simulink model "MCity_cs"  (Simulink 8.9)
settings: Solver=ode5  StartTime=0.0  StopTime=2.95  FixedStep=1/200  RelTol=1e-3
PreLoadFcn:
  | check_NUTS_defined;
  | 
  | assignin('base',['model_closed_' bdroot],false);
InitFcn:
  | PreScanExperimentInitFcn(bdroot)
StopFcn:
  | PreScanExperimentStopFcn(bdroot)
values from neighbouring files (symbols this model uses):
  d_offset = -18.15    [monocityTestLeftTurn.mat]    (also in simulation_leftTurn_PreScan.m = dl/vl*vh - 43 + R)
  vh = vhN(i)    [evaluation_leftTurn_Simulink.m]    (also in generate_leftTurn_accelerated.m = ones(N,1); generate_leftTurn_naturalistic.m = ones(N,1); monocityTestLeftTurn.mat = 30; monotonicityTest.m = i)
  vl = vlN(i)    [evaluation_leftTurn_Simulink.m]    (also in generate_leftTurn_accelerated.m = ones(N,1); generate_leftTurn_naturalistic.m = ones(N,1); monocityTestLeftTurn.mat = 60; monotonicityTest.m = j)
undefined symbols (not defined in the file or in its folder): DiscIntNeverNeededParam, warningInitialVelocity, x0
libraries: simulink x73, PreScanSimulinkLibrary x14, simulink_extras x10, PreScanUsefulBlocks x4
(part 11 of 11)

== matlab function BMW_Z3_1/MATLAB Function ==
  data: x_av input double; range output double; y_av input double; h_av_in input double; x_t input double; y_t input double; theta_worldCoordinates output double; h_av output double; theta_sensorCoordinates output double
function [range,theta_worldCoordinates,h_av,theta_sensorCoordinates] = fcn(x_av,y_av,h_av_in,x_t,y_t)
    
    range = norm([x_av-x_t,y_av-y_t]);
    theta_worldCoordinates = atan2(x_t-x_av,y_t-y_av)*180/pi;
    h_av = h_av_in;
    theta_sensorCoordinates = ((theta_worldCoordinates-h_av)*pi/180);
    theta_sensorCoordinates = mod(theta_sensorCoordinates + pi,2*pi) - pi;
    theta_sensorCoordinates = theta_sensorCoordinates/pi*180;
end

== matlab function BMW_Z3_1/Subsystem/PreBraking Model/Straight road segment/Relative velocity1/Translation ==
  data: v input double; xpd input double; xp_dot output double; TISdet parameter double
function xp_dot = trans(v, xpd, TISdet)
%#codegen
%Translation of the value

xp_dot = xpd;
for i = 1 : TISdet(1)
    if xpd(i) == v
        xp_dot(i) = 0;
    end
end
end

== matlab function BMW_Z3_1/Subsystem/PreBraking Model/Straight road segment/Relative velocity1/Embedded MATLAB Function1 ==
  settings: updateMethod=DISCRETE
  data: r input double; yp2 output double; yp1 input double; K1 input double; K2 output double; TISdet parameter double; TISMaxRange parameter double
function [yp2, K2] = modif(r, yp1, K1, TISdet, TISMaxRange)
%#codegen
% Interpolating yp value.

K2 = K1;
yp2 = yp1;

d = 50;

% Adding point
for i = 1 : TISdet(1)
   if r(i) ~= TISMaxRange(1)
      K2(i,1:d-1) = K2(i,2:d);
      K2(i,d) = yp1(i);
   end
end

% Choosing what to take
for i = 1 : TISdet(1)
    s = 0;
    suma = 0;
    for j = 1 : 50
        if K2(i,j) ~= 0
            suma = suma + K2(i,j);
            s = s + 1;
        end
    end
    yp2(i) = suma/s;
end

% Returning, if object is not detected
for i = 1: TISdet(1)
    if r(i) == TISMaxRange(1) && yp1(i) == 0
        K2(i,:,:) = zeros(d,1);
        yp2(i) = 0;
    end    
end

== matlab function Audi_A8_1/PathFollower_Preview_1/LateralController/Calculate delta steering error/eml_delta_steering_error ==
  data: v_x_vehicle input double; v_x_vehicle_Min input double; t_Preview_LatCtrl input double; delta_steeringwheeltotal output double; v_y_vehicle input double; yawrate_vehicle input double; CorneringStiffness_Tyres_Front input double; CorneringStiffness_Tyres_Rear input double; m_vehicle_total input double; inertia_z_vehicle_total input double; e_Lat input double size=10; Pos_x_CoG_Vehicle input double; wheelbase input double; RefreshCounter parameter double
function delta_steeringwheeltotal = eml_delta_steering_error(v_x_vehicle,v_x_vehicle_Min,t_Preview_LatCtrl,v_y_vehicle,yawrate_vehicle,CorneringStiffness_Tyres_Front,CorneringStiffness_Tyres_Rear,m_vehicle_total,inertia_z_vehicle_total,e_Lat,Pos_x_CoG_Vehicle,wheelbase,RefreshCounter)

delta_steeringwheeltotal = emlfcn_delta_steering_error(v_x_vehicle,v_x_vehicle_Min,t_Preview_LatCtrl,v_y_vehicle,yawrate_vehicle,CorneringStiffness_Tyres_Front,CorneringStiffness_Tyres_Rear,m_vehicle_total,inertia_z_vehicle_total,e_Lat,Pos_x_CoG_Vehicle,wheelbase,RefreshCounter);

% end function

== matlab function BMW_Z3_1/Subsystem/PreBraking Model/Straight road segment/Relative velocity2/Embedded MATLAB Function1 ==
  data: r input double; yp2 output double; yp1 input double; K1 input double; K2 output double; TISdet parameter double; TISMaxRange parameter double
function [yp2, K2] = modif(r, yp1, K1, TISdet, TISMaxRange)
%#codegen
% Interpolating yp value.

K2 = K1;
yp2 = yp1;

d = 50;

% Adding point
for i = 1 : TISdet(2)
   if r(i) ~= 5*TISMaxRange(2) 
      K2(i,1:d-1) = K2(i,2:d);
      K2(i,d) = yp1(i);
   end
end

% Choosing what to take
for i = 1 : TISdet(2)
    s = 0;
    suma = 0;
    for j = 1 : 50
        if K2(i,j) ~= 0
            suma = suma + K2(i,j);
            s = s + 1;
        end
    end
    yp2(i) = suma/s;
end

% Returning, if object is not detected
for i = 1: TISdet(2)
    if r(i) == 30 && yp1(i) == 0
        K2(i,:,:) = zeros(d,1);
        yp2(i) = 0;
    end    
end

== matlab function BMW_Z3_1/Subsystem/PreBraking Model/Straight road segment/Relative velocity2/Translation ==
  data: v input double; xpd input double; xp_dot output double; TISdet parameter double
function xp_dot = trans(v, xpd, TISdet)
%#codegen
%Translation of the value

xp_dot = xpd;
for i = 1 : TISdet(2)
    if xpd(i) == v
        xp_dot(i) =0;
    end
end
end

== matlab function BMW_Z3_1/Subsystem/PreBraking Model/TIS1sorting_fun/Embedded MATLAB Function ==
  data: range input double; indx input double; RANGE output double; TISdet parameter double
function RANGE = dis(range, indx, TISdet)
%#codegen

RANGE = zeros(TISdet(1),1);
for i = 1 : length(indx)
    if indx(i) ~= 0
        RANGE(i) = range(indx(i));
    else
        RANGE(i) = 0;
    end
end

== matlab function BMW_Z3_1/Subsystem/PreBraking Model/Straight road segment/THETA Derivative1/Deriv correction ==
  data: th input double; thp input double; thd input double; th_dot output double; TISdet parameter double
function th_dot = stopping(th, thp, thd, TISdet)
%#codegen
% Stopping if nothing is detected.

th_dot = thd;
for i = 1 : TISdet(2)
    if (th(i)==0 && thp(i)~=0) || (th(i)~=0 && thp(i)==0)
        th_dot(i) = 0;
    end
end
end

== matlab function BMW_Z3_1/Subsystem/PreBraking Model/Straight road segment/THETA Derivative2/Deriv correction ==
  data: th input double; thp input double; thd input double; th_dot output double; TISdet parameter double
function th_dot = stopping(th, thp, thd, TISdet)
%#codegen
% Stopping if nothing is detected.

th_dot = thd;
for i = 1 : TISdet(1)
    if (th(i)==0 && thp(i)~=0) || (th(i)~=0 && thp(i)==0)
        th_dot(i) = 0;
    end
end
end

== matlab function BMW_Z3_1/Subsystem/PreBraking Model/Straight road segment/THETA Derivative2/Theta extrapolation ==
  data: r input double; th1 input double; th2 output double; thd input double; time input double; K1 input double; K2 output double; TISdet parameter double; TISMaxRange parameter double
function [th2, K2] = modif(r, th1, thd, time, K1, TISdet, TISMaxRange)
%#codegen
% Interpolating theta value.

K2 = K1;
th2 = th1;

d = 10;

% Finding points used in interpolation/extrapolation.
for i = 1 : TISdet(1)
    if thd(i) ~= 0
        K2(i,1:d-1,:) = K2(i,2:d,:);
        K2(i,  d,1) = time;
        K2(i,  d,2) = th1(i);
    end
end

% Extrapolation
for i = 1 : TISdet(1)
    j = 1;
    while j < d+1 && K2(i,j,1) == 0
        j = j + 1;
    end
    
    if j > d-2
        th2(i) = th1(i);
    else
        th2(i) = interp1(K2(i,d-2:d,1),K2(i,d-2:d,2),time,'linear','extrap');
    end
end

% Returning, if object is not detected
for i = 1: TISdet(1)
    if r(i) == TISMaxRange(1) && th1(i) == 0
        K2(i,:,:) = zeros(d,2);
        th2(i) = 0;
    end    
end

end

== matlab function BMW_Z3_1/Subsystem/PreBraking Model/Straight road segment/THETA Derivative1/Theta extrapolation ==
  data: r input double; th1 input double; th2 output double; thd input double; time input double; K1 input double; K2 output double; TISdet parameter double; TISMaxRange parameter double
function [th2, K2] = modif(r, th1, thd, time, K1, TISdet, TISMaxRange)
%#codegen
% Interpolating theta value.

K2 = K1;
th2 = th1;

d = 10;

% Finding points used in interpolation/extrapolation.
for i = 1 : TISdet(2)
    if thd(i) ~= 0
        K2(i,1:d-1,:) = K2(i,2:d,:);
        K2(i,  d,1) = time;
        K2(i,  d,2) = th1(i);
    end
end

% Extrapolation
for i = 1 : TISdet(2)
    j = 1;
    while j < d+1 && K2(i,j,1) == 0
        j = j + 1;
    end
    
    if j > d-2
        th2(i) = th1(i);
    else
        th2(i) = interp1(K2(i,d-2:d,1),K2(i,d-2:d,2),time,'linear','extrap');
    end
end

% Returning, if object is not detected
for i = 1: TISdet(2)
    if r(i) == 5*TISMaxRange(2) && th1(i) == 0
        K2(i,:,:) = zeros(d,2);
        th2(i) = 0;
    end    
end

end

== matlab function BMW_Z3_1/Subsystem/PreBraking Model/Bend road segment/T2.6/median filter/median function ==
  data: u input double; y output double; TISdet parameter double
function y = fcn(u, TISdet)
%#codegen


nr = 1;
y = zeros(TISdet(nr),1,'int16');

for kk = 1 : TISdet(nr)
    z = 0;
    w = 0;
    for ii = 0 : 2
        if u(TISdet(nr)*ii+kk) == true
            w = w + 1;
        else
            z = z + 1;
        end
    end
    
    if w > z
        y(kk) = int16(1);
    end
end

end

== matlab function BMW_Z3_1/Subsystem/PreBraking Model/Bend road segment/T1.6/median filter/median function ==
  data: u input double; y output double; TISdet parameter double
function y = fcn(u, TISdet)
%#codegen


nr = 1;
y = zeros(TISdet(nr),1,'int16');

for kk = 1 : TISdet(nr)
    z = 0;
    w = 0;
    for ii = 0 : 2
        if u(TISdet(nr)*ii+kk) == true
            w = w + 1;
        else
            z = z + 1;
        end
    end
    
    if w > z
        y(kk) = int16(1);
    end
end

end

== matlab function BMW_Z3_1/Subsystem/PreBraking Model/Straight road segment/T1.6/median filter/median function ==
  data: u input double; y output double; TISdet parameter double
function y = fcn(u, TISdet)
%#codegen


nr = 1;
y = zeros(TISdet(nr),1,'int16');

for kk = 1 : TISdet(nr)
    z = 0;
    w = 0;
    for ii = 0 : 2
        if u(TISdet(nr)*ii+kk) == true
            w = w + 1;
        else
            z = z + 1;
        end
    end
    
    if w > z
        y(kk) = int16(1);
    end
end

end

== matlab function BMW_Z3_1/Subsystem/PreBraking Model/Straight road segment/T2.6/median filter/median function ==
  data: u input double; y output double; TISdet parameter double
function y = fcn(u, TISdet)
%#codegen


nr = 1;
y = zeros(TISdet(nr),1,'int16');

for kk = 1 : TISdet(nr)
    z = 0;
    w = 0;
    for ii = 0 : 2
        if u(TISdet(nr)*ii+kk) == true
            w = w + 1;
        else
            z = z + 1;
        end
    end
    
    if w > z
        y(kk) = int16(1);
    end
end

end

== matlab function BMW_Z3_1/Subsystem/PreBraking Model/TIS1sorting_fun/Embedded MATLAB Function1 ==
  data: indx input double; THETA output double; theta input double; TISdet parameter double
function THETA = ang(indx, theta, TISdet)
%#codegen

THETA = zeros(TISdet(1),1);
for i = 1 : length(indx)
    if indx(i) ~= 0
        THETA(i) = theta(indx(i));
    else
        THETA(i) = 0;
    end
end

== matlab function BMW_Z3_1/Subsystem/PreBraking Model/TIS1sorting_fun/Embedded MATLAB Function2 ==
  data: indx input double; RANGEDOT output double; rangedot input double; TISdet parameter double
function RANGEDOT = vel(indx, rangedot, TISdet)
%#codegen

RANGEDOT = zeros(TISdet(1),1);
for i = 1 : length(indx)
    if indx(i) ~= 0
        RANGEDOT(i) = rangedot(indx(i));
    else
        RANGEDOT(i) = 0;
    end
end

== matlab function BMW_Z3_1/Subsystem/PreBraking Model/TIS1sorting_fun/MATLAB Function ==
  data: indxp input double; indx output double; range input double; TISdet parameter double
function indx = sorts(indxp, range, TISdet)
%#codegen

size = TISdet(1);

indx = indxp;

for i = 1 : size
    if ( indx(i) ~= 0 ) && ( range(i) == 0)
        indx(i) = 0;
    end
end

for i = 1 : size
    if indx(i) ~= 0
        range(i) = 0;
    end
end

for i = 1 : size
    if range(i) ~= 0
       j = 1;
       while( indx(j) )
           j = j + 1;
       end
       if j ~= size
           indx(j) = i;
       end
    end
end
indx = round(indx);
end

== matlab function BMW_Z3_1/Subsystem/PreBraking Model/TIS2sorting_fun/Embedded MATLAB Function ==
  data: range input double; indx input double; RANGE output double; TISdet parameter double
function RANGE = dis(range, indx, TISdet)
%#codegen

RANGE = zeros(TISdet(2),1);
for i = 1 : length(indx)
    if indx(i) ~= 0
        RANGE(i) = range(indx(i));
    else
        RANGE(i) = 0;
    end
end

== matlab function BMW_Z3_1/Subsystem/PreBraking Model/TIS2sorting_fun/Embedded MATLAB Function1 ==
  data: indx input double; THETA output double; theta input double; TISdet parameter double
function THETA = ang(indx, theta, TISdet)
%#codegen

THETA = zeros(TISdet(2),1);
for i = 1 : length(indx)
    if indx(i) ~= 0
        THETA(i) = theta(indx(i));
    else
        THETA(i) = 0;
    end
end

== matlab function BMW_Z3_1/Subsystem/PreBraking Model/TIS2sorting_fun/Embedded MATLAB Function2 ==
  data: indx input double; RANGEDOT output double; rangedot input double; TISdet parameter double
function RANGEDOT = vel(indx, rangedot, TISdet)
%#codegen

RANGEDOT = zeros(TISdet(2),1);
for i = 1 : length(indx)
    if indx(i) ~= 0
        RANGEDOT(i) = rangedot(indx(i));
    else
        RANGEDOT(i) = 0;
    end
end

== matlab function BMW_Z3_1/Subsystem/PreBraking Model/TIS2sorting_fun/MATLAB Function ==
  data: indxp input double; indx output double; range input double; TISdet parameter double
function indx = sorts(indxp, range, TISdet)
%#codegen

size = TISdet(2);

indx = indxp;

for i = 1 : size
    if ( indx(i) ~= 0 ) && ( range(i) == 0)
        indx(i) = 0;
    end
end

for i = 1 : size
    if indx(i) ~= 0
        range(i) = 0;
    end
end

for i = 1 : size
    if range(i) ~= 0
       j = 1;
       while( indx(j) )
           j = j + 1;
       end
       if j ~= size
           indx(j) = i;
       end
    end
end
indx = round(indx);
end

== matlab function BMW_Z3_1/MATLAB Function1 ==
  data: range input double; y output double; thetaDeg input double; thresholdRange input double; thresholdThetaDeg input double
function y = fcn(range,thetaDeg,thresholdRange,thresholdThetaDeg)

% if range < thresholdRange && abs(thetaDeg)<thresholdThetaDeg
%     y = 1;
% elseif range < 0.9
%     y = 1;
% else
%     y = 0;
% end

if range < 2
    y = 1;
else
    y = 0;
end

end
